simulink library "animation_cl"  (R2018b)
settings: Solver=VariableStepAuto  StartTime=0.0  StopTime=10.0  RelTol=1e-3
libraries: vrlib x3, eulAng2RotMat_ul x1
settings Model: Creator=mcobb  LastModifiedBy=mcobb

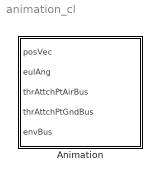
== system animation_cl ==
  Animation : Subsystem

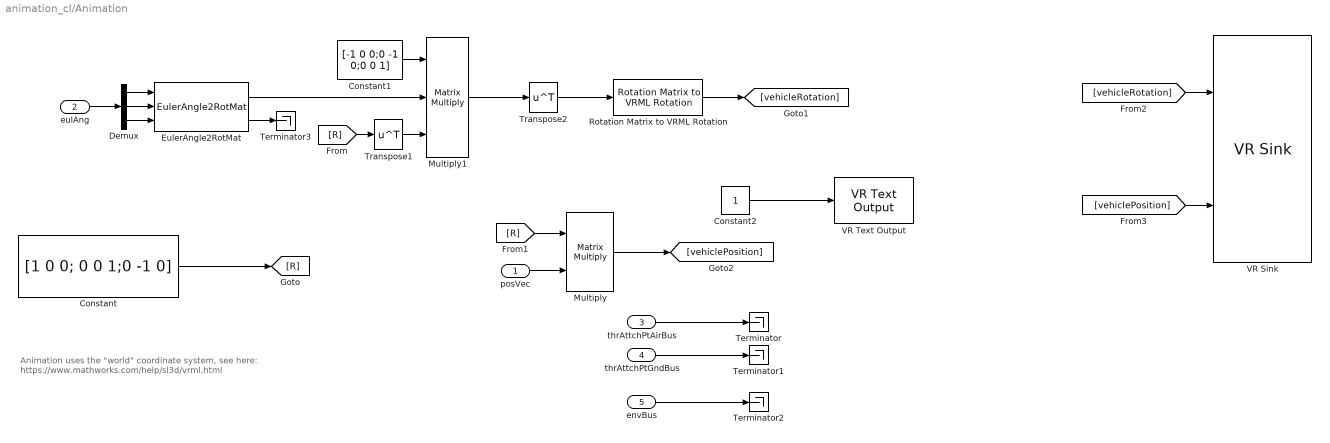
== system animation_cl/Animation ==
  note: Animation uses the "world" coordinate system, see here:
      | https://www.mathworks.com/help/sl3d/vrml.html
  posVec : Inport
  eulAng : Inport  Port=2
  thrAttchPtAirBus : Inport  Port=3
  thrAttchPtGndBus : Inport  Port=4
  envBus : Inport  Port=5
  Constant : Constant  Value=[1 0 0; 0 0 1;0 -1 0]
  Constant1 : Constant  Value=[-1 0 0;0 -1 0;0 0 1]
  Constant2 : Constant
  Demux : Demux  Outputs=3
  EulerAngle2RotMat : eulAng2RotMat_ul/EulerAngle2RotMat  SystemSampleTime=-1
  Multiply : Product  Multiplication=Matrix(*)
  Multiply1 : Product  Inputs=3  Multiplication=Matrix(*)
  Rotation Matrix to VRML Rotation : vrlib/Utilities/Rotation Matrix to VRML Rotation  maxzero=1e-12
      settings: SourceProductName=Simulink 3D Animation  SourceProductBaseCode=VR
  Terminator{,1..3} (4 alike) : Terminator
  Transpose1 : Math  Operator=transpose  SaturateOnIntegerOverflow=on
  Transpose2 : Math  Operator=transpose  SaturateOnIntegerOverflow=on
  VR Sink : vrlib/VR Sink  InstantiateOnLoad=on  SampleTime=0.1  ViewEnable=on  RemoteChange=off  RemoteView=off  FieldsWritten=Vehicle.rotation.4.1.1.double#Vehicle.translation.3.1.1.double  WorldFileName=worldFile.wrl  WorldDescription=Aerodrome in the Desert  AutoView=on  VideoDimensions=[]  AllowVariableSize=off  FigureProperties="{'Position', 'Name', 'Viewpoint', 'CameraBound', 'CameraDirection', 'CameraPosition', 'CameraUpVector', 'ZoomFactor', 'Antialiasing', 'Headlight', 'Lighting', 'NavPanel', 'Sound', 'StatusBar', 'Stereo3D', 'Stereo3DCameraOffset', 'Stereo3DHIT', 'ToolBar', 'Textures', 'Transparency', 'Triad', 'Wireframe', 'NavZones', 'NavMode', 'NavSpeed', 'CaptureFileFormat', 'CaptureFileName', 'Record2DCompressMethod', 'Record2DCompressQuality', 'Record2D', 'Record2DFileName', 'Record2DFPS'; [1.0000000000000000e+00   7.6000000000000000e+01   1.9200000000000000e+03   9.1300000000000000e+02], 'Aerodrome in the Desert', '', 'on', [1.2904010115647233e-01  -8.0041716572281141e-01   5.8538962504454162e-01], [-1.8945957183837891e+01   1.0732990264892578e+02  -5.4344623565673828e+01], [5.1850357620191700e-01   5.5765956931067084e-01   6.4820509580075059e-01], [1.0000000000000000e+00], 'on', 'on', 'on', 'halfbar', 'on', 'on', 'off', [1.0000000149011612e-01], [0.0000000000000000e+00], 'on', 'on', 'on', 'none', 'off', 'off', 'fly', 'normal', 'tif', '%f_anim_%n.tif', 'auto', [7.5000000000000000e+01], 'off', '%f_anim_%n.avi', 'auto'}"
      settings: SourceProductBaseCode=VR
  VR Text Output : vrlib/VR Text Output  Ts=-1  ForceViewerOpen=off
      settings: SourceProductName=Simulink 3D Animation  SourceProductBaseCode=VR
  wires:
  thrAttchPtAirBus/1 -> Terminator/1
  thrAttchPtGndBus/1 -> Terminator1/1
  envBus/1 -> Terminator2/1
  posVec/1 -> Multiply/2
  eulAng/1 -> Demux/1
  Multiply/1 -> [vehiclePosition]
  Demux/2 -> EulerAngle2RotMat/2
  Demux/1 -> EulerAngle2RotMat/1
  Demux/3 -> EulerAngle2RotMat/3
  EulerAngle2RotMat/1 -> Multiply1/2
  Multiply1/1 -> Transpose2/1
  Constant1/1 -> Multiply1/1
  [R] -> Multiply/1
  [vehicleRotation] -> VR Sink/1
  [vehiclePosition] -> VR Sink/2
  [R] -> Transpose1/1
  Constant/1 -> [R]
  Transpose1/1 -> Multiply1/3
  EulerAngle2RotMat/2 -> Terminator3/1
  Rotation Matrix to VRML Rotation/1 -> [vehicleRotation]
  Transpose2/1 -> Rotation Matrix to VRML Rotation/1
  Constant2/1 -> VR Text Output/1
